simulink model "FullAdder"  (R2025b)
settings: Solver=VariableStepAuto  StartTime=0.0  StopTime=10.0  RelTol=1e-3
settings Model: Creator=Soochan Kim  LastModifiedBy=Soochan Kim
settings OptimizationCC: BlockReduction=off  ConditionallyExecuteInputs=off  DefaultParameterBehavior=Inlined
settings DebuggingCC: AlgebraicLoopMsg=error
settings HardwareCC: ProdBitPerPointer=32.0  ProdBitPerSizeT=32.0  ProdBitPerPtrDiffT=32.0  ProdLargestAtomicFloat=None  ProdIntDivRoundTo=Undefined  ProdEndianess=Unspecified  ProdWordSize=32.0  ProdHWDeviceType=ASIC/FPGA->ASIC/FPGA  TargetBitPerPointer=64.0  TargetBitPerSizeT=64.0  TargetBitPerPtrDiffT=64.0  TargetLongLongMode=on  TargetIntDivRoundTo=Zero  TargetEndianess=LittleEndian  TargetWordSize=64.0  TargetHWDeviceType=Custom Processor->MATLAB Host Computer  ProdEqTarget=off

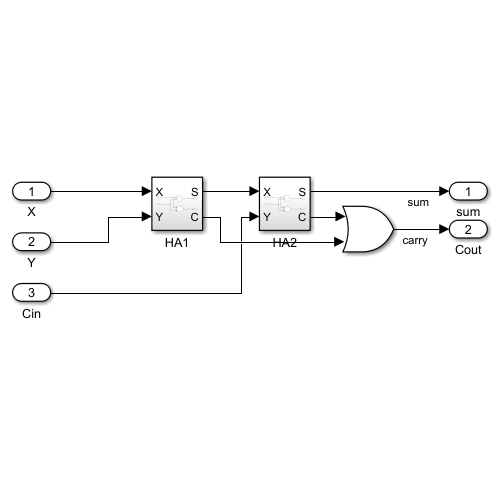
[thumbnail: Simulink's stored preview of the top-level diagram]
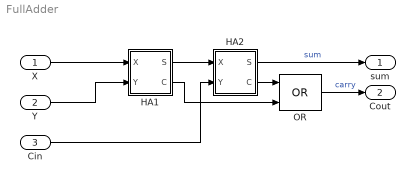
== system FullAdder ==
  X : Inport
  Y : Inport  Port=2
  Cin : Inport  Port=3
  HA1 : Subsystem
  HA2 : Subsystem
  OR : Logic  Operator=OR  IconShape=distinctive  AllPortsSameDT=off  OutDataTypeStr=boolean
  sum : Outport
  Cout : Outport  Port=2
  wires:
  HA1/1(S) -> HA2/1(X)
  OR/1 -> Cout/1  "carry"
  HA2/1(S) -> sum/1  "sum"
  HA2/2(C) -> OR/1
  Y/1 -> HA1/2(Y)
  Cin/1 -> HA2/2(Y)
  HA1/2(C) -> OR/2
  X/1 -> HA1/1(X)

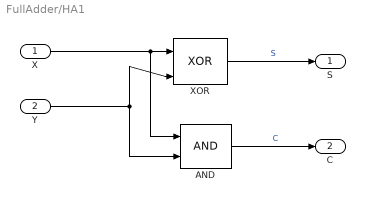
== system FullAdder/HA1 ==
  X : Inport
  Y : Inport  Port=2
  AND : Logic  IconShape=distinctive  AllPortsSameDT=off  OutDataTypeStr=boolean
  XOR : Logic  Operator=XOR  IconShape=distinctive  AllPortsSameDT=off  OutDataTypeStr=boolean
  S : Outport
  C : Outport  Port=2
  wires:
  Y/1 -> XOR/2, AND/2
  XOR/1 -> S/1  "S"
  X/1 -> AND/1, XOR/1
  AND/1 -> C/1  "C"

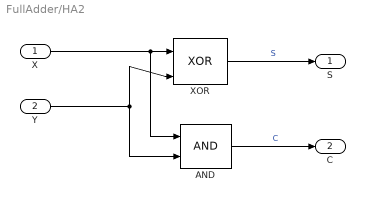
== system FullAdder/HA2 ==
  X : Inport
  Y : Inport  Port=2
  AND : Logic  IconShape=distinctive  AllPortsSameDT=off  OutDataTypeStr=boolean
  XOR : Logic  Operator=XOR  IconShape=distinctive  AllPortsSameDT=off  OutDataTypeStr=boolean
  S : Outport
  C : Outport  Port=2
  wires:
  Y/1 -> XOR/2, AND/2
  XOR/1 -> S/1  "S"
  X/1 -> AND/1, XOR/1
  AND/1 -> C/1  "C"
